simulink model "MyMotorCU_RTW"  (Simulink 10.3)
settings: Solver=ode1  StartTime=0.0  StopTime=inf  FixedStep=0.0002  RelTol=1e-3
PreLoadFcn:
  | vehicle = 'Car'; if ~length(which('cmcmd')), cmenv; end
  | MyMotorCU_RTW_bus
InitFcn:
  | vehicle = 'Car'; if ~length(which('cmcmd')), cmenv; end
  | MyMotorCU_RTW_bus
libraries: simulink x6
Description:
  | CarMaker Plug-in Model Target
settings Model: Creator=IPG  LastModifiedBy=IPG  MultithreadedSim=on
settings DataIOCC: LimitDataPoints=on
settings DebuggingCC: SFExecutionAtInitializationDiag=warning
settings HardwareCC: TargetHWDeviceType=32-bit Generic  ProdEqTarget=off
settings RTWCC: Description=CarMaker Plug-in Model Target  SystemTargetFile=CarMaker.tlc  TemplateMakefile=CarMaker_unix-linux64.tmf
settings CodeAppCC: MaxIdLength=63
settings STFCustomTargetCC: ModelReferenceCompliant=off  CodeInterfacePackaging=Reusable function  CPPClassGenCompliant=on  GRTInterface=off  GenerateAllocFcn=on  SystemTargetFile=CarMaker.tlc
settings GRTTargetCC: ModelReferenceCompliant=off  ParMdlRefBuildCompliant=off  CompOptLevelCompliant=off  ConcurrentExecutionCompliant=off  MatFileLogging=off  CodeInterfacePackaging=Reusable function  GRTInterface=off  GenerateAllocFcn=on  UseToolchainInfoCompliant=off  ExtModeMexFile=noextcomm
settings CustomProperty: DataType=string
settings EnumStrPairs: String=Car

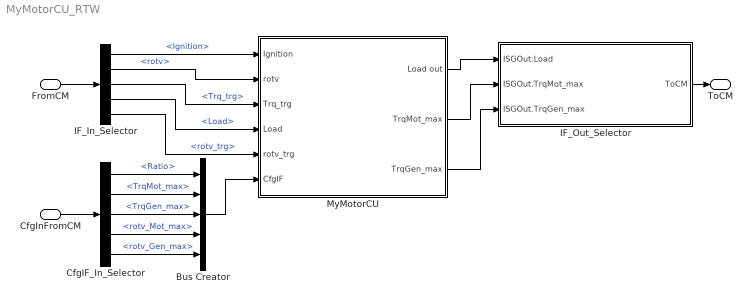
== system MyMotorCU_RTW ==
  FromCM : Inport  OutDataTypeStr=Bus: cmPTMotorCUIn
  CfgInFromCM : Inport  Port=2  OutDataTypeStr=Bus: cmPTMotorCUCfgIn
  Bus Creator : BusCreator  Inputs=5
  CfgIF_In_Selector : BusSelector  OutputSignals=ISG.Ratio,ISG.TrqMot_max,ISG.TrqGen_max,ISG.rotv_Mot_max,ISG.rotv_Gen_max
  IF_In_Selector : BusSelector  OutputSignals=Ignition,ISGIn.rotv,ISGIn.Trq_trg,ISGOut.Load,ISGIn.rotv_trg
  IF_Out_Selector : Subsystem  mask(Signal Selection){}
      mask help: Signal Selection Block
      settings: OpenFcn=cmSignalSelect('SignalSelection_CB',gcb)
  MyMotorCU : Subsystem
  ToCM : Outport  OutDataTypeStr=Bus: cmPTMotorCUOut  VectorParamsAs1DForOutWhenUnconnected=off
  wires:
  FromCM/1 -> IF_In_Selector/1
  IF_Out_Selector/1(ToCM) -> ToCM/1
  CfgInFromCM/1 -> CfgIF_In_Selector/1
  MyMotorCU/1(Load out) -> IF_Out_Selector/1(ISGOut.Load)
  MyMotorCU/2(TrqMot_max) -> IF_Out_Selector/2(ISGOut.TrqMot_max)
  MyMotorCU/3(TrqGen_max) -> IF_Out_Selector/3(ISGOut.TrqGen_max)
  IF_In_Selector/1 -> MyMotorCU/1(Ignition)  "<Ignition>"
  IF_In_Selector/2 -> MyMotorCU/2(rotv)  "<rotv>"
  IF_In_Selector/3 -> MyMotorCU/3(Trq_trg)  "<Trq_trg>"
  IF_In_Selector/4 -> MyMotorCU/4(Load)  "<Load>"
  IF_In_Selector/5 -> MyMotorCU/5(rotv_trg)  "<rotv_trg>"
  Bus Creator/1 -> MyMotorCU/6(CfgIF)
  CfgIF_In_Selector/1 -> Bus Creator/1  "<Ratio>"
  CfgIF_In_Selector/2 -> Bus Creator/2  "<TrqMot_max>"
  CfgIF_In_Selector/3 -> Bus Creator/3  "<TrqGen_max>"
  CfgIF_In_Selector/4 -> Bus Creator/4  "<rotv_Mot_max>"
  CfgIF_In_Selector/5 -> Bus Creator/5  "<rotv_Gen_max>"

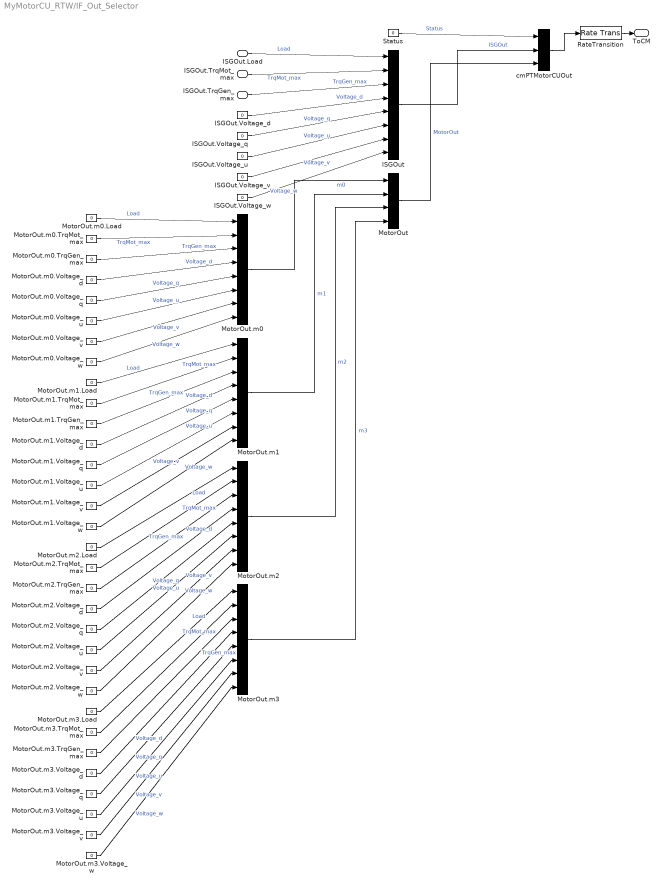
== system MyMotorCU_RTW/IF_Out_Selector ==
  ISGOut.Load : Inport
  ISGOut.TrqMot_max : Inport  Port=2
  ISGOut.TrqGen_max : Inport  Port=3
  ISGOut : BusCreator  Inputs=8
  ISGOut.Voltage_d : Constant  Value=0
  ISGOut.Voltage_q : Constant  Value=0
  ISGOut.Voltage_u : Constant  Value=0
  ISGOut.Voltage_v : Constant  Value=0
  ISGOut.Voltage_w : Constant  Value=0
  MotorOut : BusCreator  Inputs=4
  MotorOut.m{0..3} (4 alike) : BusCreator  Inputs=8
  MotorOut.m0.Load : Constant  Value=0
  MotorOut.m0.TrqGen_max : Constant  Value=0
  MotorOut.m0.TrqMot_max : Constant  Value=0
  MotorOut.m0.Voltage_d : Constant  Value=0
  MotorOut.m0.Voltage_q : Constant  Value=0
  MotorOut.m0.Voltage_u : Constant  Value=0
  MotorOut.m0.Voltage_v : Constant  Value=0
  MotorOut.m0.Voltage_w : Constant  Value=0
  MotorOut.m1.Load : Constant  Value=0
  MotorOut.m1.TrqGen_max : Constant  Value=0
  MotorOut.m1.TrqMot_max : Constant  Value=0
  MotorOut.m1.Voltage_d : Constant  Value=0
  MotorOut.m1.Voltage_q : Constant  Value=0
  MotorOut.m1.Voltage_u : Constant  Value=0
  MotorOut.m1.Voltage_v : Constant  Value=0
  MotorOut.m1.Voltage_w : Constant  Value=0
  MotorOut.m2.Load : Constant  Value=0
  MotorOut.m2.TrqGen_max : Constant  Value=0
  MotorOut.m2.TrqMot_max : Constant  Value=0
  MotorOut.m2.Voltage_d : Constant  Value=0
  MotorOut.m2.Voltage_q : Constant  Value=0
  MotorOut.m2.Voltage_u : Constant  Value=0
  MotorOut.m2.Voltage_v : Constant  Value=0
  MotorOut.m2.Voltage_w : Constant  Value=0
  MotorOut.m3.Load : Constant  Value=0
  MotorOut.m3.TrqGen_max : Constant  Value=0
  MotorOut.m3.TrqMot_max : Constant  Value=0
  MotorOut.m3.Voltage_d : Constant  Value=0
  MotorOut.m3.Voltage_q : Constant  Value=0
  MotorOut.m3.Voltage_u : Constant  Value=0
  MotorOut.m3.Voltage_v : Constant  Value=0
  MotorOut.m3.Voltage_w : Constant  Value=0
  RateTransition : RateTransition  OutPortSampleTime=str2num(get_param(bdroot,'FixedStep'))
  Status : Constant  Value=0
  cmPTMotorCUOut : BusCreator  Inputs=3
  ToCM : Outport
  wires:
  RateTransition/1 -> ToCM/1
  cmPTMotorCUOut/1 -> RateTransition/1
  Status/1 -> cmPTMotorCUOut/1  "Status"
  ISGOut/1 -> cmPTMotorCUOut/2  "ISGOut"
  ISGOut.Voltage_d/1 -> ISGOut/4  "Voltage_d"
  ISGOut.Voltage_q/1 -> ISGOut/5  "Voltage_q"
  ISGOut.Voltage_u/1 -> ISGOut/6  "Voltage_u"
  ISGOut.Voltage_v/1 -> ISGOut/7  "Voltage_v"
  ISGOut.Voltage_w/1 -> ISGOut/8  "Voltage_w"
  MotorOut/1 -> cmPTMotorCUOut/3  "MotorOut"
  MotorOut.m0/1 -> MotorOut/1  "m0"
  MotorOut.m0.Load/1 -> MotorOut.m0/1  "Load"
  MotorOut.m0.TrqMot_max/1 -> MotorOut.m0/2  "TrqMot_max"
  MotorOut.m0.TrqGen_max/1 -> MotorOut.m0/3  "TrqGen_max"
  MotorOut.m0.Voltage_d/1 -> MotorOut.m0/4  "Voltage_d"
  MotorOut.m0.Voltage_q/1 -> MotorOut.m0/5  "Voltage_q"
  MotorOut.m0.Voltage_u/1 -> MotorOut.m0/6  "Voltage_u"
  MotorOut.m0.Voltage_v/1 -> MotorOut.m0/7  "Voltage_v"
  MotorOut.m0.Voltage_w/1 -> MotorOut.m0/8  "Voltage_w"
  MotorOut.m1/1 -> MotorOut/2  "m1"
  MotorOut.m1.Load/1 -> MotorOut.m1/1  "Load"
  MotorOut.m1.TrqMot_max/1 -> MotorOut.m1/2  "TrqMot_max"
  MotorOut.m1.TrqGen_max/1 -> MotorOut.m1/3  "TrqGen_max"
  MotorOut.m1.Voltage_d/1 -> MotorOut.m1/4  "Voltage_d"
  MotorOut.m1.Voltage_q/1 -> MotorOut.m1/5  "Voltage_q"
  MotorOut.m1.Voltage_u/1 -> MotorOut.m1/6  "Voltage_u"
  MotorOut.m1.Voltage_v/1 -> MotorOut.m1/7  "Voltage_v"
  MotorOut.m1.Voltage_w/1 -> MotorOut.m1/8  "Voltage_w"
  MotorOut.m2/1 -> MotorOut/3  "m2"
  MotorOut.m2.Load/1 -> MotorOut.m2/1  "Load"
  MotorOut.m2.TrqMot_max/1 -> MotorOut.m2/2  "TrqMot_max"
  MotorOut.m2.TrqGen_max/1 -> MotorOut.m2/3  "TrqGen_max"
  MotorOut.m2.Voltage_d/1 -> MotorOut.m2/4  "Voltage_d"
  MotorOut.m2.Voltage_q/1 -> MotorOut.m2/5  "Voltage_q"
  MotorOut.m2.Voltage_u/1 -> MotorOut.m2/6  "Voltage_u"
  MotorOut.m2.Voltage_v/1 -> MotorOut.m2/7  "Voltage_v"
  MotorOut.m2.Voltage_w/1 -> MotorOut.m2/8  "Voltage_w"
  MotorOut.m3/1 -> MotorOut/4  "m3"
  MotorOut.m3.Load/1 -> MotorOut.m3/1  "Load"
  MotorOut.m3.TrqMot_max/1 -> MotorOut.m3/2  "TrqMot_max"
  MotorOut.m3.TrqGen_max/1 -> MotorOut.m3/3  "TrqGen_max"
  MotorOut.m3.Voltage_d/1 -> MotorOut.m3/4  "Voltage_d"
  MotorOut.m3.Voltage_q/1 -> MotorOut.m3/5  "Voltage_q"
  MotorOut.m3.Voltage_u/1 -> MotorOut.m3/6  "Voltage_u"
  MotorOut.m3.Voltage_v/1 -> MotorOut.m3/7  "Voltage_v"
  MotorOut.m3.Voltage_w/1 -> MotorOut.m3/8  "Voltage_w"
  ISGOut.Load/1 -> ISGOut/1  "Load"
  ISGOut.TrqMot_max/1 -> ISGOut/2  "TrqMot_max"
  ISGOut.TrqGen_max/1 -> ISGOut/3  "TrqGen_max"

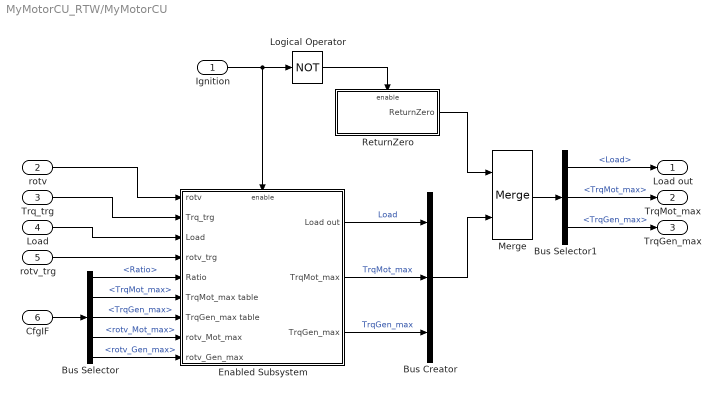
== system MyMotorCU_RTW/MyMotorCU ==
  Ignition : Inport
  rotv : Inport  Port=2
  Trq_trg : Inport  Port=3
  Load : Inport  Port=4
  rotv_trg : Inport  Port=5
  CfgIF : Inport  Port=6
  Bus Creator : BusCreator  Inputs=3
  Bus Selector : BusSelector  OutputSignals=Ratio,TrqMot_max,TrqGen_max,rotv_Mot_max,rotv_Gen_max
  Bus Selector1 : BusSelector  OutputSignals=Load,TrqMot_max,TrqGen_max
  Enabled Subsystem : Subsystem  TreatAsAtomicUnit=on
  Logical Operator : Logic  Operator=NOT  AllPortsSameDT=off  OutDataTypeStr=boolean
  Merge : Merge
  ReturnZero : Subsystem  TreatAsAtomicUnit=on
  Load out : Outport  VectorParamsAs1DForOutWhenUnconnected=off
  TrqMot_max : Outport  Port=2  VectorParamsAs1DForOutWhenUnconnected=off
  TrqGen_max : Outport  Port=3  VectorParamsAs1DForOutWhenUnconnected=off
  wires:
  Ignition/1 -> Enabled Subsystem/Enable, Logical Operator/1
  Logical Operator/1 -> ReturnZero/Enable
  rotv/1 -> Enabled Subsystem/1(rotv)
  CfgIF/1 -> Bus Selector/1
  Bus Selector/1 -> Enabled Subsystem/5(Ratio)  "<Ratio>"
  Bus Selector/2 -> Enabled Subsystem/6(TrqMot_max table)  "<TrqMot_max>"
  Bus Selector/3 -> Enabled Subsystem/7(TrqGen_max table)  "<TrqGen_max>"
  Bus Selector/4 -> Enabled Subsystem/8(rotv_Mot_max)  "<rotv_Mot_max>"
  Bus Selector/5 -> Enabled Subsystem/9(rotv_Gen_max)  "<rotv_Gen_max>"
  Trq_trg/1 -> Enabled Subsystem/2(Trq_trg)
  Load/1 -> Enabled Subsystem/3(Load)
  rotv_trg/1 -> Enabled Subsystem/4(rotv_trg)
  Enabled Subsystem/1(Load out) -> Bus Creator/1  "Load"
  Enabled Subsystem/2(TrqMot_max) -> Bus Creator/2  "TrqMot_max"
  Enabled Subsystem/3(TrqGen_max) -> Bus Creator/3  "TrqGen_max"
  ReturnZero/1(ReturnZero) -> Merge/1
  Bus Creator/1 -> Merge/2
  Merge/1 -> Bus Selector1/1
  Bus Selector1/3 -> TrqGen_max/1  "<TrqGen_max>"
  Bus Selector1/2 -> TrqMot_max/1  "<TrqMot_max>"
  Bus Selector1/1 -> Load out/1  "<Load>"

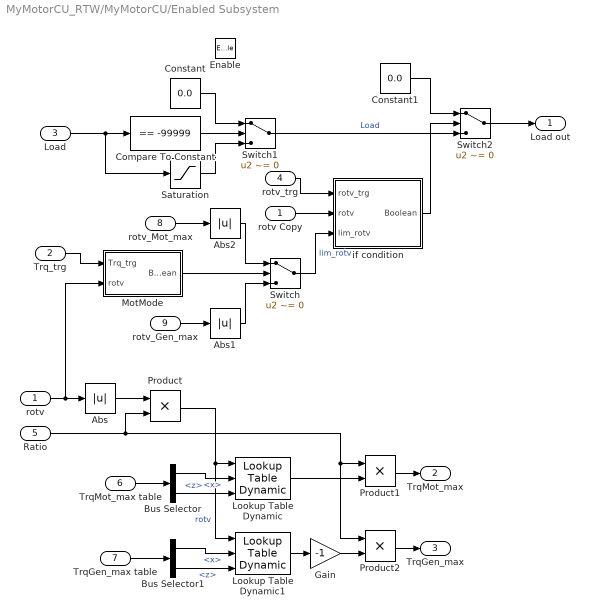
== system MyMotorCU_RTW/MyMotorCU/Enabled Subsystem ==
  rotv : Inport
  Trq_trg : Inport  Port=2
  Load : Inport  Port=3
  rotv_trg : Inport  Port=4
  Ratio : Inport  Port=5
  TrqMot_max table : Inport  Port=6
  TrqGen_max table : Inport  Port=7
  rotv_Mot_max : Inport  Port=8
  rotv_Gen_max : Inport  Port=9
  Enable : EnablePort
  Abs : Abs
  Abs1 : Abs
  Abs2 : Abs
  Bus Selector : BusSelector  OutputSignals=x,z
  Bus Selector1 : BusSelector  OutputSignals=x,z
  Compare To Constant : simulink/Logic and Bit Operations/Compare To Constant  relop===  const=-99999  OutDataTypeStr=uint8  ZeroCross=off
  Constant : Constant  Value=0.0
  Constant1 : Constant  Value=0.0
  Gain : Gain  Gain=-1
  Lookup Table Dynamic : simulink/Lookup Tables/Lookup Table Dynamic  LookUpMeth=Interpolation-Use End Values  OutDataType=float('double')  OutScaling=[]  OutputDataTypeScalingMode=Specify via dialog  OutDataTypeStr=float('double')  DoSatur=off
  Lookup Table Dynamic1 : simulink/Lookup Tables/Lookup Table Dynamic  LookUpMeth=Interpolation-Use End Values  OutDataType=float('double')  OutScaling=[]  OutputDataTypeScalingMode=Specify via dialog  OutDataTypeStr=float('double')  DoSatur=off
  MotMode : Subsystem
  Product : Product  RndMeth=Zero
  Product1 : Product  RndMeth=Zero
  Product2 : Product  RndMeth=Zero
  Saturation : Saturate  UpperLimit=1  LowerLimit=-1
  Switch : Switch  Criteria=u2 ~= 0
  Switch1 : Switch  Criteria=u2 ~= 0
  Switch2 : Switch  Criteria=u2 ~= 0
  if condition : Subsystem
  rotv Copy : InportShadow
  Load out : Outport  VectorParamsAs1DForOutWhenUnconnected=off
  TrqMot_max : Outport  Port=2  VectorParamsAs1DForOutWhenUnconnected=off
  TrqGen_max : Outport  Port=3  VectorParamsAs1DForOutWhenUnconnected=off
  wires:
  rotv/1 -> Abs/1, MotMode/2(rotv)
  Ratio/1 -> Product/2, Product2/1, Product1/1
  Abs/1 -> Product/1
  TrqMot_max table/1 -> Bus Selector/1
  Bus Selector/1 -> Lookup Table Dynamic/2  "<x>"
  TrqGen_max table/1 -> Bus Selector1/1
  Bus Selector1/1 -> Lookup Table Dynamic1/2  "<x>"
  Bus Selector1/2 -> Lookup Table Dynamic1/3  "<z>"
  Lookup Table Dynamic1/1 -> Gain/1
  rotv_Gen_max/1 -> Abs1/1
  rotv_Mot_max/1 -> Abs2/1
  Switch/1 -> if condition/3(lim_rotv)  "lim_rotv"
  Product1/1 -> TrqMot_max/1
  Product2/1 -> TrqGen_max/1
  Gain/1 -> Product2/2
  MotMode/1(Boolean) -> Switch/2
  Trq_trg/1 -> MotMode/1(Trq_trg)
  Load/1 -> Compare To Constant/1, Saturation/1
  Compare To Constant/1 -> Switch1/2
  Constant/1 -> Switch1/1
  Saturation/1 -> Switch1/3
  Switch2/1 -> Load out/1
  Constant1/1 -> Switch2/1
  Switch1/1 -> Switch2/3  "Load"
  if condition/1(Boolean) -> Switch2/2
  rotv_trg/1 -> if condition/1(rotv_trg)
  Product/1 -> Lookup Table Dynamic/1, Lookup Table Dynamic1/1  "rotv"
  Abs1/1 -> Switch/3
  Abs2/1 -> Switch/1
  Lookup Table Dynamic/1 -> Product1/2
  Bus Selector/2 -> Lookup Table Dynamic/3  "<z>"
  rotv Copy/1 -> if condition/2(rotv)

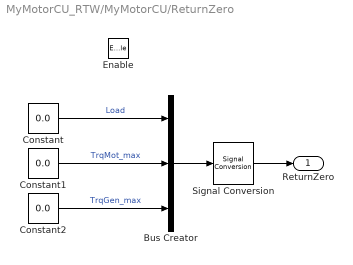
== system MyMotorCU_RTW/MyMotorCU/ReturnZero ==
  Enable : EnablePort
  Bus Creator : BusCreator  Inputs=3
  Constant : Constant  Value=0.0
  Constant1 : Constant  Value=0.0
  Constant2 : Constant  Value=0.0
  Signal Conversion : SignalConversion  ConversionOutput=Bus copy  OverrideOpt=off
  ReturnZero : Outport  VectorParamsAs1DForOutWhenUnconnected=off
  wires:
  Bus Creator/1 -> Signal Conversion/1
  Constant/1 -> Bus Creator/1  "Load"
  Constant1/1 -> Bus Creator/2  "TrqMot_max"
  Constant2/1 -> Bus Creator/3  "TrqGen_max"
  Signal Conversion/1 -> ReturnZero/1

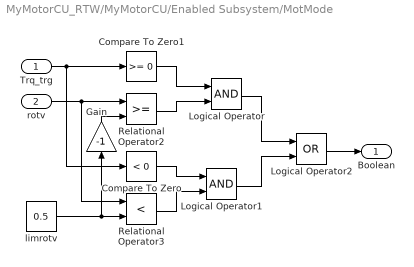
== system MyMotorCU_RTW/MyMotorCU/Enabled Subsystem/MotMode ==
  Trq_trg : Inport
  rotv : Inport  Port=2
  Compare To Zero : simulink/Logic and Bit Operations/Compare To Zero  relop=<  OutDataTypeStr=uint8  ZeroCross=off
  Compare To Zero1 : simulink/Logic and Bit Operations/Compare To Zero  relop=>=  OutDataTypeStr=uint8  ZeroCross=off
  Gain : Gain  Gain=-1
  Logical Operator : Logic  AllPortsSameDT=off  OutDataTypeStr=boolean
  Logical Operator1 : Logic  AllPortsSameDT=off  OutDataTypeStr=boolean
  Logical Operator2 : Logic  Operator=OR  AllPortsSameDT=off  OutDataTypeStr=boolean
  Relational Operator2 : RelationalOperator  OutDataTypeStr=boolean  RndMeth=Nearest
  Relational Operator3 : RelationalOperator  Operator=<  OutDataTypeStr=boolean  RndMeth=Nearest
  limrotv : Constant  Value=0.5
  Boolean : Outport  VectorParamsAs1DForOutWhenUnconnected=off
  wires:
  Logical Operator2/1 -> Boolean/1
  Logical Operator/1 -> Logical Operator2/1
  Logical Operator1/1 -> Logical Operator2/2
  Compare To Zero1/1 -> Logical Operator/1
  Trq_trg/1 -> Compare To Zero1/1, Compare To Zero/1
  Compare To Zero/1 -> Logical Operator1/1
  Relational Operator2/1 -> Logical Operator/2
  rotv/1 -> Relational Operator2/1, Relational Operator3/1
  limrotv/1 -> Relational Operator3/2, Gain/1
  Relational Operator3/1 -> Logical Operator1/2
  Gain/1 -> Relational Operator2/2

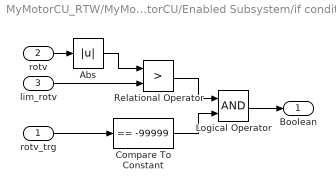
== system MyMotorCU_RTW/MyMotorCU/Enabled Subsystem/if condition ==
  rotv_trg : Inport
  rotv : Inport  Port=2
  lim_rotv : Inport  Port=3
  Abs : Abs
  Compare To Constant : simulink/Logic and Bit Operations/Compare To Constant  relop===  const=-99999  OutDataTypeStr=boolean  ZeroCross=off
  Logical Operator : Logic  AllPortsSameDT=off  OutDataTypeStr=boolean
  Relational Operator : RelationalOperator  Operator=>  OutDataTypeStr=boolean  RndMeth=Nearest
  Boolean : Outport  VectorParamsAs1DForOutWhenUnconnected=off
  wires:
  Logical Operator/1 -> Boolean/1
  rotv_trg/1 -> Compare To Constant/1
  Compare To Constant/1 -> Logical Operator/2
  Relational Operator/1 -> Logical Operator/1
  lim_rotv/1 -> Relational Operator/2
  rotv/1 -> Abs/1
  Abs/1 -> Relational Operator/1
